simulink model "lyapunov11"  (R2015b)
settings: Solver=ode4  StartTime=0.0  StopTime=50  FixedStep=0.001  RelTol=1e-3
values from neighbouring files (symbols this model uses):
  a = 0.3    [RunLyapunov11.m]
  kth = 6    [RunLyapunov11.m]
  kx = 1    [RunLyapunov11.m]
  ky = 5    [RunLyapunov11.m]
  R = 2    [RunLyapunov11.m]
  r = 0.1    [RunLyapunov11.m]
  theta0 = pi    (= 3.14159265359)    [RunLyapunov11.m]
  wd = 0.5    [RunLyapunov11.m]
  x0 = 2.3    [RunLyapunov11.m]
  y0 = 0    [RunLyapunov11.m]
settings Model: Creator=smishra  LastModifiedBy=Subodh
settings DataIOCC: LimitDataPoints=off  SaveFormat=Array
settings HardwareCC: ProdBitPerPointer=32  ProdLargestAtomicFloat=None  ProdIntDivRoundTo=Undefined  ProdEndianess=Unspecified  ProdWordSize=32  ProdHWDeviceType=32-bit Generic
settings GRTTargetCC: GeneratePreprocessorConditionals=Disable all
settings ConfigComp: CovModelRefEnable=Off

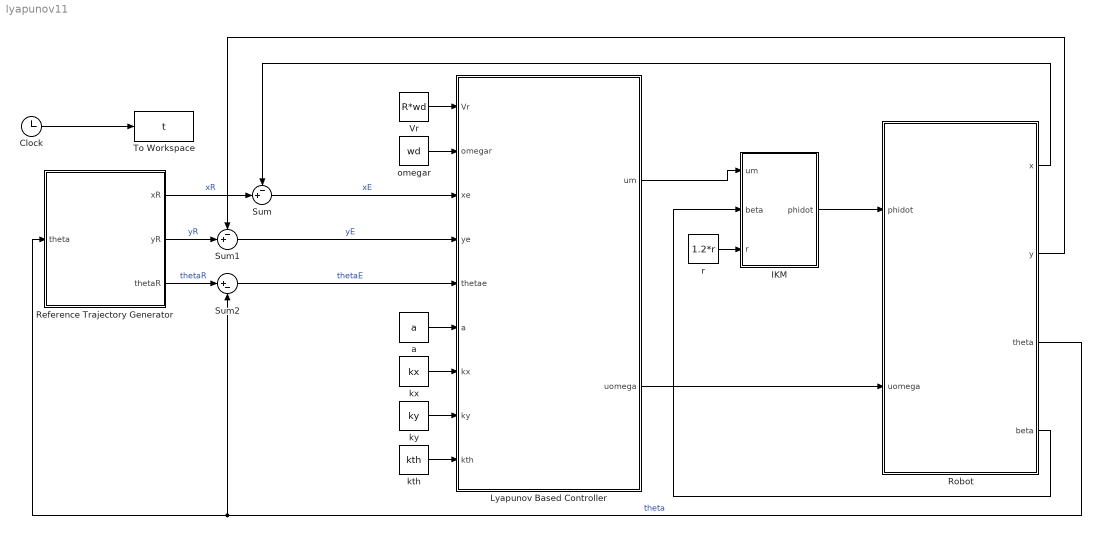
== system lyapunov11 ==
  Clock : Clock
  IKM : MATLAB Function  TreatAsAtomicUnit=on
  Lyapunov Based Controller : MATLAB Function  TreatAsAtomicUnit=on
  Reference Trajectory Generator : Subsystem
  Robot : Subsystem
  Sum : Sum  Inputs=-+|
  Sum1 : Sum  Inputs=-+|
  Sum2 : Sum  Inputs=|+-
  To Workspace : ToWorkspace  VariableName=t  SampleTime=-1
  Vr : Constant  Value=R*wd
  a : Constant  Value=a
  kth : Constant  Value=kth
  kx : Constant  Value=kx
  ky : Constant  Value=ky
  omegar : Constant  Value=wd
  r : Constant  Value=1.2*r
  wires:
  Vr/1 -> Lyapunov Based Controller/1(Vr)
  omegar/1 -> Lyapunov Based Controller/2(omegar)
  a/1 -> Lyapunov Based Controller/6(a)
  kx/1 -> Lyapunov Based Controller/7(kx)
  ky/1 -> Lyapunov Based Controller/8(ky)
  kth/1 -> Lyapunov Based Controller/9(kth)
  Reference Trajectory Generator/1(xR) -> Sum/2  "xR"
  Reference Trajectory Generator/2(yR) -> Sum1/2  "yR"
  Sum/1 -> Lyapunov Based Controller/3(xe)  "xE"
  Sum1/1 -> Lyapunov Based Controller/4(ye)  "yE"
  Sum2/1 -> Lyapunov Based Controller/5(thetae)  "thetaE"
  Clock/1 -> To Workspace/1
  Reference Trajectory Generator/3(thetaR) -> Sum2/1  "thetaR"
  Lyapunov Based Controller/2(uomega) -> Robot/2(uomega)
  IKM/1(phidot) -> Robot/1(phidot)
  Robot/4(beta) -> IKM/2(beta)
  r/1 -> IKM/3(r)
  Robot/3(theta) -> Sum2/2, Reference Trajectory Generator/1(theta)  "theta"
  Robot/1(x) -> Sum/1
  Robot/2(y) -> Sum1/1
  Lyapunov Based Controller/1(um) -> IKM/1(um)

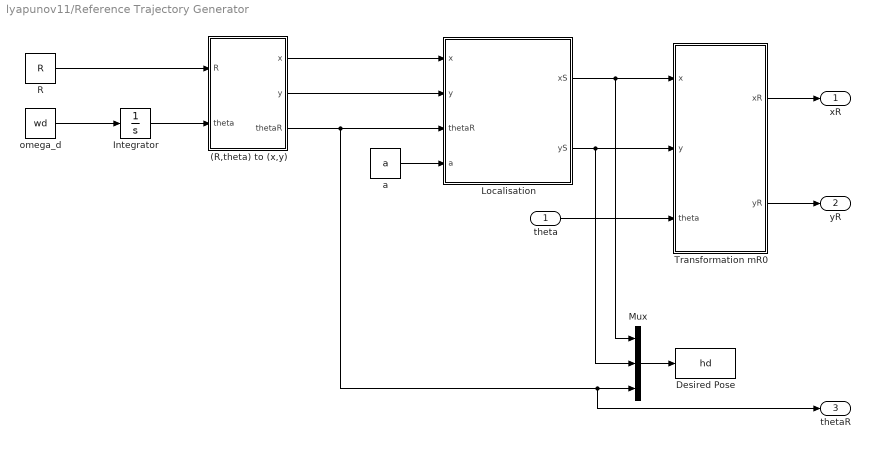
== system lyapunov11/Reference Trajectory Generator ==
  theta : Inport
  (R,theta) to (x,y) : MATLAB Function  TreatAsAtomicUnit=on
  Desired Pose : ToWorkspace  VariableName=hd  SampleTime=-1
  Integrator : Integrator
  Localisation : MATLAB Function  TreatAsAtomicUnit=on
  Mux : Mux  Inputs=3
  R : Constant  Value=R
  Transformation mR0 : MATLAB Function  TreatAsAtomicUnit=on
  a : Constant  Value=a
  omega_d : Constant  Value=wd
  xR : Outport
  yR : Outport  Port=2
  thetaR : Outport  Port=3
  wires:
  omega_d/1 -> Integrator/1
  R/1 -> (R,theta) to (x,y)/1(R)
  Integrator/1 -> (R,theta) to (x,y)/2(theta)
  Mux/1 -> Desired Pose/1
  (R,theta) to (x,y)/1(x) -> Localisation/1(x)
  (R,theta) to (x,y)/2(y) -> Localisation/2(y)
  a/1 -> Localisation/4(a)
  Localisation/1(xS) -> Transformation mR0/1(x), Mux/1
  Localisation/2(yS) -> Transformation mR0/2(y), Mux/2
  Transformation mR0/1(xR) -> xR/1
  Transformation mR0/2(yR) -> yR/1
  theta/1 -> Transformation mR0/3(theta)
  (R,theta) to (x,y)/3(thetaR) -> thetaR/1, Mux/3, Localisation/3(thetaR)

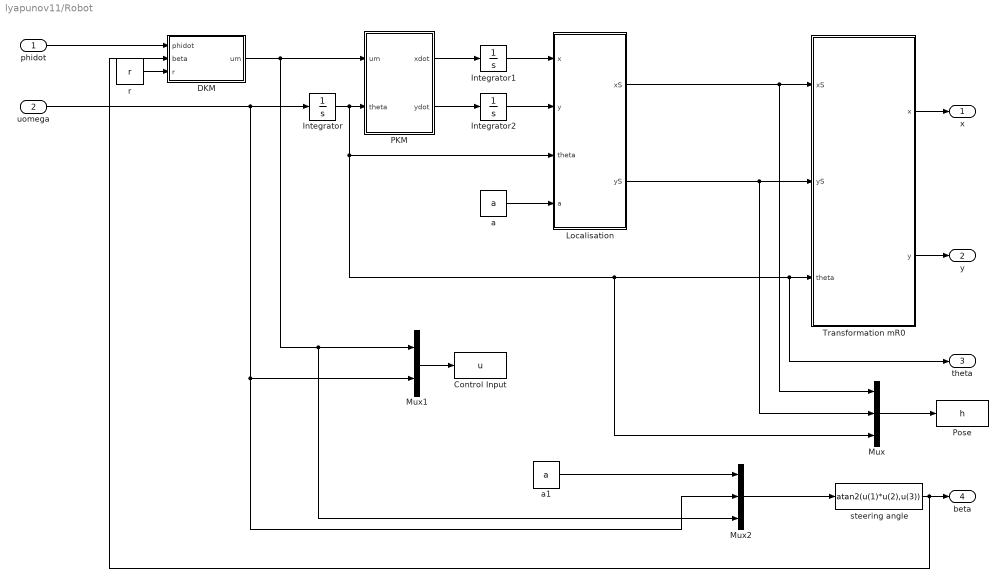
== system lyapunov11/Robot ==
  phidot : Inport
  uomega : Inport  Port=2
  Control Input : ToWorkspace  VariableName=u  SampleTime=-1
  DKM : MATLAB Function  TreatAsAtomicUnit=on
  Integrator : Integrator  InitialCondition=theta0
  Integrator1 : Integrator  InitialCondition=x0
  Integrator2 : Integrator  InitialCondition=y0
  Localisation : MATLAB Function  TreatAsAtomicUnit=on
  Mux : Mux  Inputs=3
  Mux1 : Mux  Inputs=2
  Mux2 : Mux  Inputs=3
  PKM : MATLAB Function  TreatAsAtomicUnit=on
  Pose : ToWorkspace  VariableName=h  SampleTime=-1
  Transformation mR0 : MATLAB Function  TreatAsAtomicUnit=on
  a : Constant  Value=a
  a1 : Constant  Value=a
  r : Constant  Value=r
  steering angle : Fcn  Expr=atan2(u(1)*u(2),u(3))
  x : Outport
  y : Outport  Port=2
  theta : Outport  Port=3
  beta : Outport  Port=4
  wires:
  uomega/1 -> Integrator/1, Mux2/2, Mux1/2
  PKM/1(xdot) -> Integrator1/1
  PKM/2(ydot) -> Integrator2/1
  Integrator1/1 -> Localisation/1(x)
  Integrator2/1 -> Localisation/2(y)
  a/1 -> Localisation/4(a)
  Localisation/1(xS) -> Mux/1, Transformation mR0/1(xS)
  Transformation mR0/2(y) -> y/1
  Transformation mR0/1(x) -> x/1
  Localisation/2(yS) -> Mux/2, Transformation mR0/2(yS)
  Mux/1 -> Pose/1
  Mux1/1 -> Control Input/1
  steering angle/1 -> DKM/2(beta), beta/1
  a1/1 -> Mux2/1
  phidot/1 -> DKM/1(phidot)
  DKM/1(um) -> Mux2/3, Mux1/1, PKM/1(um)
  r/1 -> DKM/3(r)
  Integrator/1 -> Mux/3, theta/1, Transformation mR0/3(theta), Localisation/3(theta), PKM/2(theta)
  Mux2/1 -> steering angle/1

== matlab function lyapunov11/Reference Trajectory Generator/Transformation mR0 ==
  data: x input; y input; theta input; xR output; yR output
function [xR,yR]= mR0(x,y,theta)
%#codegen

xR=cos(theta)*x+sin(theta)*y;
yR=-sin(theta)*x+cos(theta)*y;
end

== matlab function lyapunov11/Reference Trajectory Generator/(R,theta) to (x,y) ==
  data: x output; R input; y output; theta input; thetaR output
function [x,y,thetaR]= toCartesian(R,theta)
%#codegen

x=R*cos(theta);
y=R*sin(theta);
thetaR=theta+pi/2;
end

== matlab function lyapunov11/Robot/PKM ==
  data: um input; theta input; xdot output; ydot output
function [xdot,ydot]= PKM(um,theta)
%#codegen
xdot=um*cos(theta);
ydot=um*sin(theta);
end

== matlab function lyapunov11/Robot/Localisation ==
  data: x input; y input; theta input; xS output; yS output; a input
function [xS,yS]= Localisation(x,y,theta,a)
%#codegen
xS=x+a*cos(theta);
yS=y+a*sin(theta);
end

== matlab function lyapunov11/Robot/Transformation mR0 ==
  data: xS input; yS input; x output; y output; theta input
function [x,y]= mR0(xS,yS,theta)
%#codegen

x=cos(theta)*xS+sin(theta)*yS;
y=-sin(theta)*xS+cos(theta)*yS;
end

== matlab function lyapunov11/Lyapunov Based Controller ==
  data: Vr input; omegar input; xe input; ye input; thetae input; a input; kx input; ky input; kth input; um output; uomega output
function [um,uomega] = controller(Vr,omegar,xe,ye,thetae,a,kx,ky,kth)
%#codegen
um=Vr*cos(thetae)-omegar*a*sin(thetae)+kx*xe;
uomega=((Vr*sin(thetae)+omegar*a*cos(thetae))*ky*ye+omegar*thetae+kth*thetae^2)/(a*ky*ye+thetae);
end

== matlab function lyapunov11/Reference Trajectory Generator/Localisation ==
  data: x input; y input; thetaR input; xS output; yS output; a input
function [xS,yS]= Localisation(x,y,thetaR,a)
%#codegen
xS=x+a*cos(thetaR);
yS=y+a*sin(thetaR);
end

== matlab function lyapunov11/IKM ==
  data: um input; beta input; phidot output; r input
function phidot = IKM(um,beta,r)
%#codegen
phidot=(1/(r*cos(beta)))*um;
end

== matlab function lyapunov11/Robot/DKM ==
  data: phidot input; um output; beta input; r input
function um = DKM(phidot,beta,r)
%#codegen
um=r*cos(beta)*phidot;
end
